simulink model "fuzzyPDpart2"  (R2025b)
settings: Solver=VariableStepAuto  StartTime=0.0  StopTime=300  RelTol=1e-3
libraries: fuzblock x1

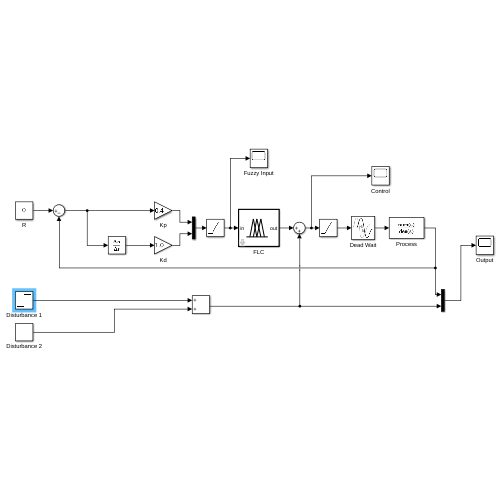
[thumbnail: Simulink's stored preview of the top-level diagram]
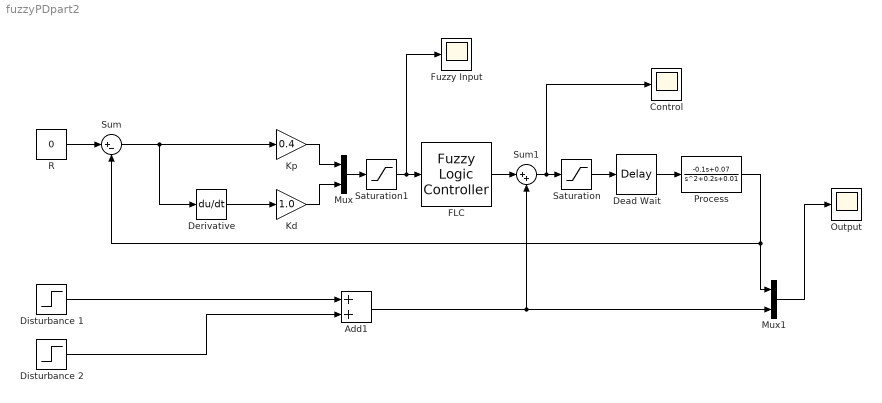
== system fuzzyPDpart2 ==
  Add1 : Sum
  Control : Scope
      settings: ActiveDisplayYMinimum=-1.5546580150348959  ActiveDisplayYMaximum=1.3481482578092443  DataLoggingVariableName=ScopeData2
  Dead Wait : TransportDelay  DelayTime=3
  Derivative : Derivative
  Disturbance 1 : Step  Time=0  After=0.5  SampleTime=0
  Disturbance 2 : Step  Time=100  After=-1  SampleTime=0
  FLC : fuzblock/Fuzzy Logic  Controller  FIS='Copy_of_fuzzyPDmodel.fis'  OutputSampleNumber=101  DataType=double  UseLookupTable=off  NumBreakpoints=10  FuzzifiedInputs=off  RuleFiringStrengths=off  RuleOutputs=off  AggregatedOutputs=off  SimulateUsing=Interpreted execution  OutOfRangeInputValueMessage=warning  NoRuleFiredMessage=warning  EmptyOutputFuzzySetMessage=warning
  Fuzzy Input : Scope
      settings: ActiveDisplayYMinimum=-1.5546580150348959  ActiveDisplayYMaximum=1.3481482578092443
  Kd : Gain  Gain=1.0
  Kp : Gain  Gain=0.4
  Mux : Mux  Inputs=2
  Mux1 : Mux  Inputs=2
  Output : Scope
      settings: ActiveDisplayYMinimum=-1.5546580150348959  ActiveDisplayYMaximum=1.3481482578092443
  Process : TransferFcn  Numerator=[-0.1 0.07]  Denominator=[1 0.2 0.01]
  R : Constant  Value=0
  Saturation : Saturate  UpperLimit=1.0  LowerLimit=-1.0
  Saturation1 : Saturate  UpperLimit=1.0  LowerLimit=-1.0
  Sum : Sum  Inputs=|+-
  Sum1 : Sum  Inputs=|++
  wires:
  Sum/1 -> Kp/1, Derivative/1
  Kp/1 -> Mux/1
  Kd/1 -> Mux/2
  Derivative/1 -> Kd/1
  Process/1 -> Mux1/1, Sum/2
  Dead Wait/1 -> Process/1
  Saturation/1 -> Dead Wait/1
  R/1 -> Sum/1
  Sum1/1 -> Control/1, Saturation/1
  FLC/1 -> Sum1/1
  Add1/1 -> Sum1/2, Mux1/2
  Mux1/1 -> Output/1
  Disturbance 1/1 -> Add1/1
  Disturbance 2/1 -> Add1/2
  Mux/1 -> Saturation1/1
  Saturation1/1 -> Fuzzy Input/1, FLC/1
